simulink model "My_Model"  (R2022a)
settings: Solver=VariableStepAuto  StartTime=0.0  StopTime=10.0  RelTol=1e-3
libraries: neural x1294, spsSeriesRLCBranchLib x16, spsDiodeLib x14, spsMosfetLib x9, spsVoltageMeasurementLib x9, powerlib_extras x8, spsThreePhaseVIMeasurementLib x7, spsCurrentMeasurementLib x4, spsPVArrayLib x4, spsPWMGeneratorDCDCLib x4, spsTHDLib x4, spsThreePhaseParallelRLCBranchLib x3
(part 41 of 41)

== system My_Model/VSC Control/Current Regulator/7 layer network/Layer 6/LW{6,4} ==
  "ad{6,4}" : Inport  PortDimensions=25
      mask Display: e = 0.06;c1 = [120 230 180]/255;c2 = ([120 230 180]+0)/(256+128);c3 = ([120 230 180]+128)/(256+128);patch([0 1 1 0],[0 0 1 1],c1);patch([0 1 1 1-e 1-e 0+e],[0 0 1 1-e 0+e 0+e],c2);patch([0 0 1 1-e 0+e 0+e],[0 1 1 1-e 1-e 0+e],c3);plot([0 1 1 0 0],[0 0 1 1 0]);
  "IW{6,4}(1,:)'" : Constant  Value=[-0.377172170865255840244145701944944448769092559814453125;0.2166215985231878249361869848144124262034893035888671875;-0.8493855795188680612994858165620826184749603271484375;0.43917994402737026149452503887005150318145751953125;0.9925973529188081290186573824030347168445587158203125;0.52191832200732390933950455291778780519962310791015625;0.54353768542801095264849209343083202838897705078125;0.275162210381826144445227555479505099356174468994140625;0.81569668151233631903096465975977480411529541015625;-0.93565711696775666350589517605840228497982025146484375;-0.95509797101199678248661939505836926400661468505859375;0.09267489111664718726135703263935283757746219635009765625;-0.957854254009712580142377191805280745029449462890625;0.9681511422261415145129603843088261783123016357421875;0.59514371716452518779050251396256498992443084716796875;0.752293859537388254210554805467836558818817138671875;0.71189958405266562380120376474224030971527099609375;0.43163356736211000441727492216159589588642120361328125;-0.48098452705637051440845652905409224331378936767578125;-0.5182102404330437561696953707723878324031829833984375;-0.76663173461491995741567961886175908148288726806640625;0.920833310401809601586364806280471384525299072265625;-0.470710370173132275350980080474982969462871551513671875;-0.291630162894867428491352256969548761844635009765625;-0.363147996214426560523946818648255430161952972412109375]
      mask Display: e = 0.06;c1 = [120 150 230]/255;c2 = ([120 150 230]+0)/383;c3 = ([120 150 230]+128)/383;patch([0 1 1 0],[0 0 1 1],c1);patch([0 1 1 1-e 1-e 0+e],[0 0 1 1-e 0+e 0+e],c2);patch([0 0 1 1-e 0+e 0+e],[0 1 1 1-e 1-e 0+e],c3);plot([0 1 1 0 0],[0 0 1 1 0]);disp('weights');
  "IW{6,4}(2,:)'" : Constant  Value=[0.28732507639288284995160438484163023531436920166015625;-0.10063068272491536292445601930012344382703304290771484375;-0.07588109417358383790297438054039957933127880096435546875;0.8685538436173725340694318219902925193309783935546875;0.6786737694400650777737382668419741094112396240234375;0.034625140595084556716098944662007852457463741302490234375;-0.283134669546071748857940519883413799107074737548828125;0.08902086054486742228153417499925126321613788604736328125;-1.0830744519321864327565663188579492270946502685546875;0.1886613708921636434201474230576422996819019317626953125;0.71261338952339248198342147588846273720264434814453125;0.481217533055725843471606140155927278101444244384765625;0.311161297820213011977585892964270897209644317626953125;0.04995362741111118720649386659715673886239528656005859375;0.94351257987673953220308931122417561709880828857421875;0.66959181319910410223883445723913609981536865234375;0.7286748401637630490057517818058840930461883544921875;0.693751372005718902613580212346278131008148193359375;0.429237930795354827306908873651991598308086395263671875;0.432163392727505757395789487418369390070438385009765625;0.19340272304600369945859483777894638478755950927734375;-0.0179994719843084016730472285416908562183380126953125;1.1024282588912923674939747797907330095767974853515625;-0.413702287461697515436043204317684285342693328857421875;0.9039180203867420715369007666595280170440673828125]
      mask Display: e = 0.06;c1 = [120 150 230]/255;c2 = ([120 150 230]+0)/383;c3 = ([120 150 230]+128)/383;patch([0 1 1 0],[0 0 1 1],c1);patch([0 1 1 1-e 1-e 0+e],[0 0 1 1-e 0+e 0+e],c2);patch([0 0 1 1-e 0+e 0+e],[0 1 1 1-e 1-e 0+e],c3);plot([0 1 1 0 0],[0 0 1 1 0]);disp('weights');
  "IW{6,4}(3,:)'" : Constant  Value=[-0.64629750703306065862108198416535742580890655517578125;-1.098756912740348479218255306477658450603485107421875;-0.08866746573161542188667993968920200131833553314208984375;-1.07761686120664013088799038087017834186553955078125;-0.08707633180751157830901121315037016756832599639892578125;-0.69038565434756959948714438723982311785221099853515625;1.0878215450123225327416776053723879158496856689453125;0.35531945282508503591856197090237401425838470458984375;-0.469159418146348039524440309833153150975704193115234375;0.3372642338873126366394217257038690149784088134765625;0.08822785475541576605262861221490311436355113983154296875;1.1142599806591240163555767139769159257411956787109375;0.72730830477476182682750049934838898479938507080078125;1.0873952419514834044633744269958697259426116943359375;0.69099352817197712273156184892286546528339385986328125;-0.53374420227049845788513948718900792300701141357421875;0.1658638052207602464616087445392622612416744232177734375;-0.11318910522164206400308472666438319720327854156494140625;0.97839969428519679706113265638123266398906707763671875;-0.88106106612810630718257698390516452491283416748046875;-1.0220826746153062192234983740490861237049102783203125;0.3896164522899236981601234219851903617382049560546875;-1.0826724324468883775551830694894306361675262451171875;-0.87968776248958013841416914146975614130496978759765625;-0.0002833283639702526002235316582300583831965923309326171875]
      mask Display: e = 0.06;c1 = [120 150 230]/255;c2 = ([120 150 230]+0)/383;c3 = ([120 150 230]+128)/383;patch([0 1 1 0],[0 0 1 1],c1);patch([0 1 1 1-e 1-e 0+e],[0 0 1 1-e 0+e 0+e],c2);patch([0 0 1 1-e 0+e 0+e],[0 1 1 1-e 1-e 0+e],c3);plot([0 1 1 0 0],[0 0 1 1 0]);disp('weights');
  "IW{6,4}(4,:)'" : Constant  Value=[0.1890485194098358856518160564519348554313182830810546875;0.0216342621174379808046683848488100920803844928741455078125;0.12011949005118673083902791631771833635866641998291015625;-0.7077852872841623455002491027698852121829986572265625;-0.422049459183063968570337465280317701399326324462890625;-0.1909842843294208003523948491420014761388301849365234375;-1.1988173017738776859886229431140236556529998779296875;0.556276063052497438121690720436163246631622314453125;-0.79012741190201729590825152627076022326946258544921875;0.3767786001003521345609215131844393908977508544921875;0.4643024120214291894370717272977344691753387451171875;-0.1428330266733211229013278398269903846085071563720703125;0.468537774485975722082997663164860568940639495849609375;-1.0556031236689114027882396840141154825687408447265625;-0.50465636007393721573777156663709320127964019775390625;-0.67913261552524406550190860798466019332408905029296875;0.172008584272319298147380095542757771909236907958984375;-0.144475965090768265763898625664296559989452362060546875;1.001598299104828004857381529291160404682159423828125;-0.93051931461395931410862658594851382076740264892578125;0.796164649884228747822589866700582206249237060546875;0.96609541574008073183676970074884593486785888671875;-0.440361911057138843972325048525817692279815673828125;1.01609392982572810382180250599049031734466552734375;0.28456750588627055531532050736132077872753143310546875]
      mask Display: e = 0.06;c1 = [120 150 230]/255;c2 = ([120 150 230]+0)/383;c3 = ([120 150 230]+128)/383;patch([0 1 1 0],[0 0 1 1],c1);patch([0 1 1 1-e 1-e 0+e],[0 0 1 1-e 0+e 0+e],c2);patch([0 0 1 1-e 0+e 0+e],[0 1 1 1-e 1-e 0+e],c3);plot([0 1 1 0 0],[0 0 1 1 0]);disp('weights');
  "IW{6,4}(5,:)'" : Constant  Value=[0.27105149658062133166680496287881396710872650146484375;-0.193023461694903641916454262172919698059558868408203125;0.7128488109947801465438033119426108896732330322265625;-0.07239340949961368953946561077827936969697475433349609375;-0.9830308857488956331138751920661889016628265380859375;-0.7342459118544735208189422337454743683338165283203125;0.76633670396205888497576097506680525839328765869140625;-0.91777628549413592384809135182877071201801300048828125;0.99199765136458928349583175076986663043498992919921875;0.86263812078303647723487301846034824848175048828125;-0.642325683690944782000542545574717223644256591796875;-0.92113551914019320410176305813365615904331207275390625;-0.322276526479408131908854784342111088335514068603515625;-0.66431651873548169806582563978736288845539093017578125;-0.781701747176127614835650092572905123233795166015625;-0.39731852184941807148987891196156851947307586669921875;-0.461111000145560334662064860822283662855625152587890625;-0.059668897380601833291269286974056740291416645050048828125;0.55032218363215446021996513081830926239490509033203125;-0.70264903726413774354142560696345753967761993408203125;0.50662619166864775177572255415725521743297576904296875;0.09871715719628242069472179309741477482020854949951171875;1.0938888762767418061372381998808123171329498291015625;-0.80978778041068510962219306748011149466037750244140625;0.1924043984401257734173640301378327421844005584716796875]
      mask Display: e = 0.06;c1 = [120 150 230]/255;c2 = ([120 150 230]+0)/383;c3 = ([120 150 230]+128)/383;patch([0 1 1 0],[0 0 1 1],c1);patch([0 1 1 1-e 1-e 0+e],[0 0 1 1-e 0+e 0+e],c2);patch([0 0 1 1-e 0+e 0+e],[0 1 1 1-e 1-e 0+e],c3);plot([0 1 1 0 0],[0 0 1 1 0]);disp('weights');
  Mux : Mux  Inputs=5
      mask Display: e = 0.06;c1 = [120 150 230]/255;c2 = ([120 150 230]+0)/383;c3 = ([120 150 230]+128)/383;patch([0 1 1 0],[0 0 1 1],c1);patch([0 1 1 1-e 1-e 0+e],[0 0 1 1-e 0+e 0+e],c2);patch([0 0 1 1-e 0+e 0+e],[0 1 1 1-e 1-e 0+e],c3);plot([0 1 1 0 0],[0 0 1 1 0]);disp('Mux');
  dotprod{1..5} (5 alike) : neural/Weight Functions/dotprod
  "lz{6,4}" : Outport
      mask Display: e = 0.06;c1 = [120 230 180]/255;c2 = ([120 230 180]+0)/(256+128);c3 = ([120 230 180]+128)/(256+128);patch([0 1 1 0],[0 0 1 1],c1);patch([0 1 1 1-e 1-e 0+e],[0 0 1 1-e 0+e 0+e],c2);patch([0 0 1 1-e 0+e 0+e],[0 1 1 1-e 1-e 0+e],c3);plot([0 1 1 0 0],[0 0 1 1 0]);
  wires:
  "IW{6,4}(1,:)'"/1 -> dotprod1/1
  "ad{6,4}"/1 -> dotprod1/2, dotprod2/2, dotprod3/2, dotprod4/2, dotprod5/2
  dotprod1/1 -> Mux/1
  "IW{6,4}(2,:)'"/1 -> dotprod2/1
  dotprod2/1 -> Mux/2
  "IW{6,4}(3,:)'"/1 -> dotprod3/1
  dotprod3/1 -> Mux/3
  "IW{6,4}(4,:)'"/1 -> dotprod4/1
  dotprod4/1 -> Mux/4
  "IW{6,4}(5,:)'"/1 -> dotprod5/1
  dotprod5/1 -> Mux/5
  Mux/1 -> "lz{6,4}"/1

== system My_Model/VSC Control/Current Regulator/7 layer network/Layer 6/LW{6,5} ==
  "ad{6,5}" : Inport  PortDimensions=10
      mask Display: e = 0.06;c1 = [120 230 180]/255;c2 = ([120 230 180]+0)/(256+128);c3 = ([120 230 180]+128)/(256+128);patch([0 1 1 0],[0 0 1 1],c1);patch([0 1 1 1-e 1-e 0+e],[0 0 1 1-e 0+e 0+e],c2);patch([0 0 1 1-e 0+e 0+e],[0 1 1 1-e 1-e 0+e],c3);plot([0 1 1 0 0],[0 0 1 1 0]);
  "IW{6,5}(1,:)'" : Constant  Value=[0.429687815971328934683270972527679987251758575439453125;-0.346068629113729875346194830854074098169803619384765625;-0.98219313699815113949398437398485839366912841796875;-0.83739498807844869876504390049376524984836578369140625;-0.7885264055381722148041490072500891983509063720703125;-0.8543528519776548701969431931502185761928558349609375;0.035004635751464806270316643121986999176442623138427734375;-1.039210679049491492520473912009038031101226806640625;0.34006931875280965726915383129380643367767333984375;-0.502979274986845581452143960632383823394775390625]
      mask Display: e = 0.06;c1 = [120 150 230]/255;c2 = ([120 150 230]+0)/383;c3 = ([120 150 230]+128)/383;patch([0 1 1 0],[0 0 1 1],c1);patch([0 1 1 1-e 1-e 0+e],[0 0 1 1-e 0+e 0+e],c2);patch([0 0 1 1-e 0+e 0+e],[0 1 1 1-e 1-e 0+e],c3);plot([0 1 1 0 0],[0 0 1 1 0]);disp('weights');
  "IW{6,5}(2,:)'" : Constant  Value=[-1.0710077128761394948952556660515256226062774658203125;0.80353619826974165274435790706775151193141937255859375;-0.98744244173064676939333139671362005174160003662109375;0.68583647556494942154614591345307417213916778564453125;0.6769723731389734044938677470781840384006500244140625;0.8110004105230468329779114355915226042270660400390625;-0.38681250645933251686159337623394094407558441162109375;1.0558527284464924722584555638604797422885894775390625;-0.481185456649400100648250599988386966288089752197265625;0.56609801374014845354309954927884973585605621337890625]
      mask Display: e = 0.06;c1 = [120 150 230]/255;c2 = ([120 150 230]+0)/383;c3 = ([120 150 230]+128)/383;patch([0 1 1 0],[0 0 1 1],c1);patch([0 1 1 1-e 1-e 0+e],[0 0 1 1-e 0+e 0+e],c2);patch([0 0 1 1-e 0+e 0+e],[0 1 1 1-e 1-e 0+e],c3);plot([0 1 1 0 0],[0 0 1 1 0]);disp('weights');
  "IW{6,5}(3,:)'" : Constant  Value=[0.06271534584953468438595081124731223098933696746826171875;-0.57758435101291649704791097974521107971668243408203125;-1.1214217969680639885865502947126515209674835205078125;0.287195615160836414947453931745258159935474395751953125;-0.9518543521969726750597828868194483220577239990234375;0.49129271852601552605932511141872964799404144287109375;0.39119008942367405889939391272491775453090667724609375;1.1269337522951523578029764394159428775310516357421875;0.60893532118659077223554731972399167716503143310546875;0.9641221714535419540226257595350034534931182861328125]
      mask Display: e = 0.06;c1 = [120 150 230]/255;c2 = ([120 150 230]+0)/383;c3 = ([120 150 230]+128)/383;patch([0 1 1 0],[0 0 1 1],c1);patch([0 1 1 1-e 1-e 0+e],[0 0 1 1-e 0+e 0+e],c2);patch([0 0 1 1-e 0+e 0+e],[0 1 1 1-e 1-e 0+e],c3);plot([0 1 1 0 0],[0 0 1 1 0]);disp('weights');
  "IW{6,5}(4,:)'" : Constant  Value=[-1.158415351011949478987617112579755485057830810546875;0.1915558214143078530344865839651902206242084503173828125;0.444350035799105536060693566469126380980014801025390625;-1.0584621783405434580771498076501302421092987060546875;-0.6575764228372922293175406593945808708667755126953125;0.57266541551685989919207031562109477818012237548828125;-0.9518889867230029278033498485456220805644989013671875;-0.92910349289341065404101982494466938078403472900390625;0.13672757324302164949614279976231046020984649658203125;0.557587726090502666664860953460447490215301513671875]
      mask Display: e = 0.06;c1 = [120 150 230]/255;c2 = ([120 150 230]+0)/383;c3 = ([120 150 230]+128)/383;patch([0 1 1 0],[0 0 1 1],c1);patch([0 1 1 1-e 1-e 0+e],[0 0 1 1-e 0+e 0+e],c2);patch([0 0 1 1-e 0+e 0+e],[0 1 1 1-e 1-e 0+e],c3);plot([0 1 1 0 0],[0 0 1 1 0]);disp('weights');
  "IW{6,5}(5,:)'" : Constant  Value=[0.74460524721355880739537269619177095592021942138671875;0.99773442819647539803185054552159272134304046630859375;0.212480488677939838293440288907731883227825164794921875;-0.97662617042054578053722480035503394901752471923828125;-0.56627909108300344964703754158108495175838470458984375;0.341773472356023566565141891260282136499881744384765625;-0.79744639055360144741513295230106450617313385009765625;-0.0739957191774893996427664433213067241013050079345703125;-0.1541052068468630464881385933040292002260684967041015625;-0.1981364354380889258866460522767738439142704010009765625]
      mask Display: e = 0.06;c1 = [120 150 230]/255;c2 = ([120 150 230]+0)/383;c3 = ([120 150 230]+128)/383;patch([0 1 1 0],[0 0 1 1],c1);patch([0 1 1 1-e 1-e 0+e],[0 0 1 1-e 0+e 0+e],c2);patch([0 0 1 1-e 0+e 0+e],[0 1 1 1-e 1-e 0+e],c3);plot([0 1 1 0 0],[0 0 1 1 0]);disp('weights');
  Mux : Mux  Inputs=5
      mask Display: e = 0.06;c1 = [120 150 230]/255;c2 = ([120 150 230]+0)/383;c3 = ([120 150 230]+128)/383;patch([0 1 1 0],[0 0 1 1],c1);patch([0 1 1 1-e 1-e 0+e],[0 0 1 1-e 0+e 0+e],c2);patch([0 0 1 1-e 0+e 0+e],[0 1 1 1-e 1-e 0+e],c3);plot([0 1 1 0 0],[0 0 1 1 0]);disp('Mux');
  dotprod{1..5} (5 alike) : neural/Weight Functions/dotprod
  "lz{6,5}" : Outport
      mask Display: e = 0.06;c1 = [120 230 180]/255;c2 = ([120 230 180]+0)/(256+128);c3 = ([120 230 180]+128)/(256+128);patch([0 1 1 0],[0 0 1 1],c1);patch([0 1 1 1-e 1-e 0+e],[0 0 1 1-e 0+e 0+e],c2);patch([0 0 1 1-e 0+e 0+e],[0 1 1 1-e 1-e 0+e],c3);plot([0 1 1 0 0],[0 0 1 1 0]);
  wires:
  "IW{6,5}(1,:)'"/1 -> dotprod1/1
  "ad{6,5}"/1 -> dotprod1/2, dotprod2/2, dotprod3/2, dotprod4/2, dotprod5/2
  dotprod1/1 -> Mux/1
  "IW{6,5}(2,:)'"/1 -> dotprod2/1
  dotprod2/1 -> Mux/2
  "IW{6,5}(3,:)'"/1 -> dotprod3/1
  dotprod3/1 -> Mux/3
  "IW{6,5}(4,:)'"/1 -> dotprod4/1
  dotprod4/1 -> Mux/4
  "IW{6,5}(5,:)'"/1 -> dotprod5/1
  dotprod5/1 -> Mux/5
  Mux/1 -> "lz{6,5}"/1

== system My_Model/VSC Control/Current Regulator/7 layer network/Layer 7/Delays 1 ==
  "p{7}" : Inport  PortDimensions=2
      mask Display: e = 0.06;c1 = [120 230 180]/255;c2 = ([120 230 180]+0)/(256+128);c3 = ([120 230 180]+128)/(256+128);patch([0 1 1 0],[0 0 1 1],c1);patch([0 1 1 1-e 1-e 0+e],[0 0 1 1-e 0+e 0+e],c2);patch([0 0 1 1-e 0+e 0+e],[0 1 1 1-e 1-e 0+e],c3);plot([0 1 1 0 0],[0 0 1 1 0]);
  mux : Mux  Inputs=1
      mask Display: e = 0.06;c1 = [120 150 230]/255;c2 = ([120 150 230]+0)/383;c3 = ([120 150 230]+128)/383;patch([0 1 1 0],[0 0 1 1],c1);patch([0 1 1 1-e 1-e 0+e],[0 0 1 1-e 0+e 0+e],c2);patch([0 0 1 1-e 0+e 0+e],[0 1 1 1-e 1-e 0+e],c3);plot([0 1 1 0 0],[0 0 1 1 0]);disp('Mux')
  "pd{7,1}" : Outport
      mask Display: e = 0.06;c1 = [120 230 180]/255;c2 = ([120 230 180]+0)/(256+128);c3 = ([120 230 180]+128)/(256+128);patch([0 1 1 0],[0 0 1 1],c1);patch([0 1 1 1-e 1-e 0+e],[0 0 1 1-e 0+e 0+e],c2);patch([0 0 1 1-e 0+e 0+e],[0 1 1 1-e 1-e 0+e],c3);plot([0 1 1 0 0],[0 0 1 1 0]);
  wires:
  "p{7}"/1 -> mux/1
  mux/1 -> "pd{7,1}"/1

== system My_Model/VSC Control/Current Regulator/7 layer network/Layer 7/Delays 2 ==
  "p{7}" : Inport  PortDimensions=5
      mask Display: e = 0.06;c1 = [120 230 180]/255;c2 = ([120 230 180]+0)/(256+128);c3 = ([120 230 180]+128)/(256+128);patch([0 1 1 0],[0 0 1 1],c1);patch([0 1 1 1-e 1-e 0+e],[0 0 1 1-e 0+e 0+e],c2);patch([0 0 1 1-e 0+e 0+e],[0 1 1 1-e 1-e 0+e],c3);plot([0 1 1 0 0],[0 0 1 1 0]);
  mux : Mux  Inputs=1
      mask Display: e = 0.06;c1 = [120 150 230]/255;c2 = ([120 150 230]+0)/383;c3 = ([120 150 230]+128)/383;patch([0 1 1 0],[0 0 1 1],c1);patch([0 1 1 1-e 1-e 0+e],[0 0 1 1-e 0+e 0+e],c2);patch([0 0 1 1-e 0+e 0+e],[0 1 1 1-e 1-e 0+e],c3);plot([0 1 1 0 0],[0 0 1 1 0]);disp('Mux')
  "pd{7,1}" : Outport
      mask Display: e = 0.06;c1 = [120 230 180]/255;c2 = ([120 230 180]+0)/(256+128);c3 = ([120 230 180]+128)/(256+128);patch([0 1 1 0],[0 0 1 1],c1);patch([0 1 1 1-e 1-e 0+e],[0 0 1 1-e 0+e 0+e],c2);patch([0 0 1 1-e 0+e 0+e],[0 1 1 1-e 1-e 0+e],c3);plot([0 1 1 0 0],[0 0 1 1 0]);
  wires:
  "p{7}"/1 -> mux/1
  mux/1 -> "pd{7,1}"/1

== system My_Model/VSC Control/Current Regulator/7 layer network/Layer 7/Delays 3 ==
  "p{7}" : Inport  PortDimensions=10
      mask Display: e = 0.06;c1 = [120 230 180]/255;c2 = ([120 230 180]+0)/(256+128);c3 = ([120 230 180]+128)/(256+128);patch([0 1 1 0],[0 0 1 1],c1);patch([0 1 1 1-e 1-e 0+e],[0 0 1 1-e 0+e 0+e],c2);patch([0 0 1 1-e 0+e 0+e],[0 1 1 1-e 1-e 0+e],c3);plot([0 1 1 0 0],[0 0 1 1 0]);
  mux : Mux  Inputs=1
      mask Display: e = 0.06;c1 = [120 150 230]/255;c2 = ([120 150 230]+0)/383;c3 = ([120 150 230]+128)/383;patch([0 1 1 0],[0 0 1 1],c1);patch([0 1 1 1-e 1-e 0+e],[0 0 1 1-e 0+e 0+e],c2);patch([0 0 1 1-e 0+e 0+e],[0 1 1 1-e 1-e 0+e],c3);plot([0 1 1 0 0],[0 0 1 1 0]);disp('Mux')
  "pd{7,2}" : Outport
      mask Display: e = 0.06;c1 = [120 230 180]/255;c2 = ([120 230 180]+0)/(256+128);c3 = ([120 230 180]+128)/(256+128);patch([0 1 1 0],[0 0 1 1],c1);patch([0 1 1 1-e 1-e 0+e],[0 0 1 1-e 0+e 0+e],c2);patch([0 0 1 1-e 0+e 0+e],[0 1 1 1-e 1-e 0+e],c3);plot([0 1 1 0 0],[0 0 1 1 0]);
  wires:
  "p{7}"/1 -> mux/1
  mux/1 -> "pd{7,2}"/1

== system My_Model/VSC Control/Current Regulator/7 layer network/Layer 7/Delays 4 ==
  "p{7}" : Inport  PortDimensions=20
      mask Display: e = 0.06;c1 = [120 230 180]/255;c2 = ([120 230 180]+0)/(256+128);c3 = ([120 230 180]+128)/(256+128);patch([0 1 1 0],[0 0 1 1],c1);patch([0 1 1 1-e 1-e 0+e],[0 0 1 1-e 0+e 0+e],c2);patch([0 0 1 1-e 0+e 0+e],[0 1 1 1-e 1-e 0+e],c3);plot([0 1 1 0 0],[0 0 1 1 0]);
  mux : Mux  Inputs=1
      mask Display: e = 0.06;c1 = [120 150 230]/255;c2 = ([120 150 230]+0)/383;c3 = ([120 150 230]+128)/383;patch([0 1 1 0],[0 0 1 1],c1);patch([0 1 1 1-e 1-e 0+e],[0 0 1 1-e 0+e 0+e],c2);patch([0 0 1 1-e 0+e 0+e],[0 1 1 1-e 1-e 0+e],c3);plot([0 1 1 0 0],[0 0 1 1 0]);disp('Mux')
  "pd{7,3}" : Outport
      mask Display: e = 0.06;c1 = [120 230 180]/255;c2 = ([120 230 180]+0)/(256+128);c3 = ([120 230 180]+128)/(256+128);patch([0 1 1 0],[0 0 1 1],c1);patch([0 1 1 1-e 1-e 0+e],[0 0 1 1-e 0+e 0+e],c2);patch([0 0 1 1-e 0+e 0+e],[0 1 1 1-e 1-e 0+e],c3);plot([0 1 1 0 0],[0 0 1 1 0]);
  wires:
  "p{7}"/1 -> mux/1
  mux/1 -> "pd{7,3}"/1

== system My_Model/VSC Control/Current Regulator/7 layer network/Layer 7/Delays 5 ==
  "p{7}" : Inport  PortDimensions=25
      mask Display: e = 0.06;c1 = [120 230 180]/255;c2 = ([120 230 180]+0)/(256+128);c3 = ([120 230 180]+128)/(256+128);patch([0 1 1 0],[0 0 1 1],c1);patch([0 1 1 1-e 1-e 0+e],[0 0 1 1-e 0+e 0+e],c2);patch([0 0 1 1-e 0+e 0+e],[0 1 1 1-e 1-e 0+e],c3);plot([0 1 1 0 0],[0 0 1 1 0]);
  mux : Mux  Inputs=1
      mask Display: e = 0.06;c1 = [120 150 230]/255;c2 = ([120 150 230]+0)/383;c3 = ([120 150 230]+128)/383;patch([0 1 1 0],[0 0 1 1],c1);patch([0 1 1 1-e 1-e 0+e],[0 0 1 1-e 0+e 0+e],c2);patch([0 0 1 1-e 0+e 0+e],[0 1 1 1-e 1-e 0+e],c3);plot([0 1 1 0 0],[0 0 1 1 0]);disp('Mux')
  "pd{7,4}" : Outport
      mask Display: e = 0.06;c1 = [120 230 180]/255;c2 = ([120 230 180]+0)/(256+128);c3 = ([120 230 180]+128)/(256+128);patch([0 1 1 0],[0 0 1 1],c1);patch([0 1 1 1-e 1-e 0+e],[0 0 1 1-e 0+e 0+e],c2);patch([0 0 1 1-e 0+e 0+e],[0 1 1 1-e 1-e 0+e],c3);plot([0 1 1 0 0],[0 0 1 1 0]);
  wires:
  "p{7}"/1 -> mux/1
  mux/1 -> "pd{7,4}"/1

== system My_Model/VSC Control/Current Regulator/7 layer network/Layer 7/Delays 6 ==
  "p{7}" : Inport  PortDimensions=10
      mask Display: e = 0.06;c1 = [120 230 180]/255;c2 = ([120 230 180]+0)/(256+128);c3 = ([120 230 180]+128)/(256+128);patch([0 1 1 0],[0 0 1 1],c1);patch([0 1 1 1-e 1-e 0+e],[0 0 1 1-e 0+e 0+e],c2);patch([0 0 1 1-e 0+e 0+e],[0 1 1 1-e 1-e 0+e],c3);plot([0 1 1 0 0],[0 0 1 1 0]);
  mux : Mux  Inputs=1
      mask Display: e = 0.06;c1 = [120 150 230]/255;c2 = ([120 150 230]+0)/383;c3 = ([120 150 230]+128)/383;patch([0 1 1 0],[0 0 1 1],c1);patch([0 1 1 1-e 1-e 0+e],[0 0 1 1-e 0+e 0+e],c2);patch([0 0 1 1-e 0+e 0+e],[0 1 1 1-e 1-e 0+e],c3);plot([0 1 1 0 0],[0 0 1 1 0]);disp('Mux')
  "pd{7,5}" : Outport
      mask Display: e = 0.06;c1 = [120 230 180]/255;c2 = ([120 230 180]+0)/(256+128);c3 = ([120 230 180]+128)/(256+128);patch([0 1 1 0],[0 0 1 1],c1);patch([0 1 1 1-e 1-e 0+e],[0 0 1 1-e 0+e 0+e],c2);patch([0 0 1 1-e 0+e 0+e],[0 1 1 1-e 1-e 0+e],c3);plot([0 1 1 0 0],[0 0 1 1 0]);
  wires:
  "p{7}"/1 -> mux/1
  mux/1 -> "pd{7,5}"/1

== system My_Model/VSC Control/Current Regulator/7 layer network/Layer 7/Delays 7 ==
  "p{7}" : Inport  PortDimensions=5
      mask Display: e = 0.06;c1 = [120 230 180]/255;c2 = ([120 230 180]+0)/(256+128);c3 = ([120 230 180]+128)/(256+128);patch([0 1 1 0],[0 0 1 1],c1);patch([0 1 1 1-e 1-e 0+e],[0 0 1 1-e 0+e 0+e],c2);patch([0 0 1 1-e 0+e 0+e],[0 1 1 1-e 1-e 0+e],c3);plot([0 1 1 0 0],[0 0 1 1 0]);
  mux : Mux  Inputs=1
      mask Display: e = 0.06;c1 = [120 150 230]/255;c2 = ([120 150 230]+0)/383;c3 = ([120 150 230]+128)/383;patch([0 1 1 0],[0 0 1 1],c1);patch([0 1 1 1-e 1-e 0+e],[0 0 1 1-e 0+e 0+e],c2);patch([0 0 1 1-e 0+e 0+e],[0 1 1 1-e 1-e 0+e],c3);plot([0 1 1 0 0],[0 0 1 1 0]);disp('Mux')
  "pd{7,6}" : Outport
      mask Display: e = 0.06;c1 = [120 230 180]/255;c2 = ([120 230 180]+0)/(256+128);c3 = ([120 230 180]+128)/(256+128);patch([0 1 1 0],[0 0 1 1],c1);patch([0 1 1 1-e 1-e 0+e],[0 0 1 1-e 0+e 0+e],c2);patch([0 0 1 1-e 0+e 0+e],[0 1 1 1-e 1-e 0+e],c3);plot([0 1 1 0 0],[0 0 1 1 0]);
  wires:
  "p{7}"/1 -> mux/1
  mux/1 -> "pd{7,6}"/1

== system My_Model/VSC Control/Current Regulator/7 layer network/Layer 7/IW{7,1} ==
  "pd{7,1}" : Inport  PortDimensions=2
      mask Display: e = 0.06;c1 = [120 230 180]/255;c2 = ([120 230 180]+0)/(256+128);c3 = ([120 230 180]+128)/(256+128);patch([0 1 1 0],[0 0 1 1],c1);patch([0 1 1 1-e 1-e 0+e],[0 0 1 1-e 0+e 0+e],c2);patch([0 0 1 1-e 0+e 0+e],[0 1 1 1-e 1-e 0+e],c3);plot([0 1 1 0 0],[0 0 1 1 0]);
  "IW{7,1}(1,:)'" : Constant  Value=[1.271226380744853390325488362577743828296661376953125;-0.017924339888765794537306419442757032811641693115234375]
      mask Display: e = 0.06;c1 = [120 150 230]/255;c2 = ([120 150 230]+0)/383;c3 = ([120 150 230]+128)/383;patch([0 1 1 0],[0 0 1 1],c1);patch([0 1 1 1-e 1-e 0+e],[0 0 1 1-e 0+e 0+e],c2);patch([0 0 1 1-e 0+e 0+e],[0 1 1 1-e 1-e 0+e],c3);plot([0 1 1 0 0],[0 0 1 1 0]);disp('Weights');
  "IW{7,1}(2,:)'" : Constant  Value=[-0.253325923879466008425964673733687959611415863037109375;0.752854052452355926305926914210431277751922607421875]
      mask Display: e = 0.06;c1 = [120 150 230]/255;c2 = ([120 150 230]+0)/383;c3 = ([120 150 230]+128)/383;patch([0 1 1 0],[0 0 1 1],c1);patch([0 1 1 1-e 1-e 0+e],[0 0 1 1-e 0+e 0+e],c2);patch([0 0 1 1-e 0+e 0+e],[0 1 1 1-e 1-e 0+e],c3);plot([0 1 1 0 0],[0 0 1 1 0]);disp('Weights');
  Mux : Mux  Inputs=2
      mask Display: e = 0.06;c1 = [120 150 230]/255;c2 = ([120 150 230]+0)/383;c3 = ([120 150 230]+128)/383;patch([0 1 1 0],[0 0 1 1],c1);patch([0 1 1 1-e 1-e 0+e],[0 0 1 1-e 0+e 0+e],c2);patch([0 0 1 1-e 0+e 0+e],[0 1 1 1-e 1-e 0+e],c3);plot([0 1 1 0 0],[0 0 1 1 0]);disp('Mux');
  dotprod1 : neural/Weight Functions/dotprod
  dotprod2 : neural/Weight Functions/dotprod
  "iz{7,1}" : Outport
      mask Display: e = 0.06;c1 = [120 230 180]/255;c2 = ([120 230 180]+0)/(256+128);c3 = ([120 230 180]+128)/(256+128);patch([0 1 1 0],[0 0 1 1],c1);patch([0 1 1 1-e 1-e 0+e],[0 0 1 1-e 0+e 0+e],c2);patch([0 0 1 1-e 0+e 0+e],[0 1 1 1-e 1-e 0+e],c3);plot([0 1 1 0 0],[0 0 1 1 0]);
  wires:
  "IW{7,1}(1,:)'"/1 -> dotprod1/1
  "pd{7,1}"/1 -> dotprod1/2, dotprod2/2
  dotprod1/1 -> Mux/1
  "IW{7,1}(2,:)'"/1 -> dotprod2/1
  dotprod2/1 -> Mux/2
  Mux/1 -> "iz{7,1}"/1

== system My_Model/VSC Control/Current Regulator/7 layer network/Layer 7/LW{7,1} ==
  "ad{7,1}" : Inport  PortDimensions=5
      mask Display: e = 0.06;c1 = [120 230 180]/255;c2 = ([120 230 180]+0)/(256+128);c3 = ([120 230 180]+128)/(256+128);patch([0 1 1 0],[0 0 1 1],c1);patch([0 1 1 1-e 1-e 0+e],[0 0 1 1-e 0+e 0+e],c2);patch([0 0 1 1-e 0+e 0+e],[0 1 1 1-e 1-e 0+e],c3);plot([0 1 1 0 0],[0 0 1 1 0]);
  "IW{7,1}(1,:)'" : Constant  Value=[-0.1399721419724498094883102794483420439064502716064453125;0.9169102476718442584768808956141583621501922607421875;-0.33071053243995873760496806426090188324451446533203125;-0.60184994233361199800214080823934637010097503662109375;0.58924366070781120097166194682358764111995697021484375]
      mask Display: e = 0.06;c1 = [120 150 230]/255;c2 = ([120 150 230]+0)/383;c3 = ([120 150 230]+128)/383;patch([0 1 1 0],[0 0 1 1],c1);patch([0 1 1 1-e 1-e 0+e],[0 0 1 1-e 0+e 0+e],c2);patch([0 0 1 1-e 0+e 0+e],[0 1 1 1-e 1-e 0+e],c3);plot([0 1 1 0 0],[0 0 1 1 0]);disp('weights');
  "IW{7,1}(2,:)'" : Constant  Value=[-0.5457231422189112723941661897697485983371734619140625;-0.57571827217991222713777688113623298704624176025390625;0.1647711432619676508171124851287459023296833038330078125;0.183526978590318912143430907235597260296344757080078125;0.0237926496519859191625112515566797810606658458709716796875]
      mask Display: e = 0.06;c1 = [120 150 230]/255;c2 = ([120 150 230]+0)/383;c3 = ([120 150 230]+128)/383;patch([0 1 1 0],[0 0 1 1],c1);patch([0 1 1 1-e 1-e 0+e],[0 0 1 1-e 0+e 0+e],c2);patch([0 0 1 1-e 0+e 0+e],[0 1 1 1-e 1-e 0+e],c3);plot([0 1 1 0 0],[0 0 1 1 0]);disp('weights');
  Mux : Mux  Inputs=2
      mask Display: e = 0.06;c1 = [120 150 230]/255;c2 = ([120 150 230]+0)/383;c3 = ([120 150 230]+128)/383;patch([0 1 1 0],[0 0 1 1],c1);patch([0 1 1 1-e 1-e 0+e],[0 0 1 1-e 0+e 0+e],c2);patch([0 0 1 1-e 0+e 0+e],[0 1 1 1-e 1-e 0+e],c3);plot([0 1 1 0 0],[0 0 1 1 0]);disp('Mux');
  dotprod1 : neural/Weight Functions/dotprod
  dotprod2 : neural/Weight Functions/dotprod
  "lz{7,1}" : Outport
      mask Display: e = 0.06;c1 = [120 230 180]/255;c2 = ([120 230 180]+0)/(256+128);c3 = ([120 230 180]+128)/(256+128);patch([0 1 1 0],[0 0 1 1],c1);patch([0 1 1 1-e 1-e 0+e],[0 0 1 1-e 0+e 0+e],c2);patch([0 0 1 1-e 0+e 0+e],[0 1 1 1-e 1-e 0+e],c3);plot([0 1 1 0 0],[0 0 1 1 0]);
  wires:
  "IW{7,1}(1,:)'"/1 -> dotprod1/1
  "ad{7,1}"/1 -> dotprod1/2, dotprod2/2
  dotprod1/1 -> Mux/1
  "IW{7,1}(2,:)'"/1 -> dotprod2/1
  dotprod2/1 -> Mux/2
  Mux/1 -> "lz{7,1}"/1

== system My_Model/VSC Control/Current Regulator/7 layer network/Layer 7/LW{7,2} ==
  "ad{7,2}" : Inport  PortDimensions=10
      mask Display: e = 0.06;c1 = [120 230 180]/255;c2 = ([120 230 180]+0)/(256+128);c3 = ([120 230 180]+128)/(256+128);patch([0 1 1 0],[0 0 1 1],c1);patch([0 1 1 1-e 1-e 0+e],[0 0 1 1-e 0+e 0+e],c2);patch([0 0 1 1-e 0+e 0+e],[0 1 1 1-e 1-e 0+e],c3);plot([0 1 1 0 0],[0 0 1 1 0]);
  "IW{7,2}(1,:)'" : Constant  Value=[0.295330180327427083142310948460362851619720458984375;-0.5251128972157454999347692137234844267368316650390625;-0.7180734971715343473164239185280166566371917724609375;0.5919270243185563717958075358183123171329498291015625;0.11953399765489790274042292139711207710206508636474609375;0.342647990599721563587110040316474623978137969970703125;-0.0159771387543272691544871122459881007671356201171875;-0.704647027112888846289706634706817567348480224609375;-0.091153538469831374424501291287015192210674285888671875;-0.157429755972143536890683890305808745324611663818359375]
      mask Display: e = 0.06;c1 = [120 150 230]/255;c2 = ([120 150 230]+0)/383;c3 = ([120 150 230]+128)/383;patch([0 1 1 0],[0 0 1 1],c1);patch([0 1 1 1-e 1-e 0+e],[0 0 1 1-e 0+e 0+e],c2);patch([0 0 1 1-e 0+e 0+e],[0 1 1 1-e 1-e 0+e],c3);plot([0 1 1 0 0],[0 0 1 1 0]);disp('weights');
  "IW{7,2}(2,:)'" : Constant  Value=[0.65692183983364749177980002059484831988811492919921875;0.2333722687588110911161010108116897754371166229248046875;0.040390642172835687639942392479497357271611690521240234375;0.7737311897419905104555937214172445237636566162109375;-0.309691966896001591447173950655269436538219451904296875;0.66971479097063635332887088225106708705425262451171875;1.0306742930276191483329739639884792268276214599609375;-0.59097725639540066300270382271264679729938507080078125;0.0019314451221247551371273942777406773529946804046630859375;-0.336081037894097656160141696091159246861934661865234375]
      mask Display: e = 0.06;c1 = [120 150 230]/255;c2 = ([120 150 230]+0)/383;c3 = ([120 150 230]+128)/383;patch([0 1 1 0],[0 0 1 1],c1);patch([0 1 1 1-e 1-e 0+e],[0 0 1 1-e 0+e 0+e],c2);patch([0 0 1 1-e 0+e 0+e],[0 1 1 1-e 1-e 0+e],c3);plot([0 1 1 0 0],[0 0 1 1 0]);disp('weights');
  Mux : Mux  Inputs=2
      mask Display: e = 0.06;c1 = [120 150 230]/255;c2 = ([120 150 230]+0)/383;c3 = ([120 150 230]+128)/383;patch([0 1 1 0],[0 0 1 1],c1);patch([0 1 1 1-e 1-e 0+e],[0 0 1 1-e 0+e 0+e],c2);patch([0 0 1 1-e 0+e 0+e],[0 1 1 1-e 1-e 0+e],c3);plot([0 1 1 0 0],[0 0 1 1 0]);disp('Mux');
  dotprod1 : neural/Weight Functions/dotprod
  dotprod2 : neural/Weight Functions/dotprod
  "lz{7,2}" : Outport
      mask Display: e = 0.06;c1 = [120 230 180]/255;c2 = ([120 230 180]+0)/(256+128);c3 = ([120 230 180]+128)/(256+128);patch([0 1 1 0],[0 0 1 1],c1);patch([0 1 1 1-e 1-e 0+e],[0 0 1 1-e 0+e 0+e],c2);patch([0 0 1 1-e 0+e 0+e],[0 1 1 1-e 1-e 0+e],c3);plot([0 1 1 0 0],[0 0 1 1 0]);
  wires:
  "IW{7,2}(1,:)'"/1 -> dotprod1/1
  "ad{7,2}"/1 -> dotprod1/2, dotprod2/2
  dotprod1/1 -> Mux/1
  "IW{7,2}(2,:)'"/1 -> dotprod2/1
  dotprod2/1 -> Mux/2
  Mux/1 -> "lz{7,2}"/1

== system My_Model/VSC Control/Current Regulator/7 layer network/Layer 7/LW{7,3} ==
  "ad{7,3}" : Inport  PortDimensions=20
      mask Display: e = 0.06;c1 = [120 230 180]/255;c2 = ([120 230 180]+0)/(256+128);c3 = ([120 230 180]+128)/(256+128);patch([0 1 1 0],[0 0 1 1],c1);patch([0 1 1 1-e 1-e 0+e],[0 0 1 1-e 0+e 0+e],c2);patch([0 0 1 1-e 0+e 0+e],[0 1 1 1-e 1-e 0+e],c3);plot([0 1 1 0 0],[0 0 1 1 0]);
  "IW{7,3}(1,:)'" : Constant  Value=[0.20027745385358297625089107896201312541961669921875;-0.1260101494140383471265209891498670913279056549072265625;-0.52953910171273255169666072106338106095790863037109375;0.188971290437726036071097723834100179374217987060546875;-0.580890073741141321761460858397185802459716796875;-0.28614803792992937747641235546325333416461944580078125;0.66112637931677242786321357925771735608577728271484375;0.77887882743118230788326172842062078416347503662109375;0.486831181941093316112301181419752538204193115234375;0.86114110403958876727159577058046124875545501708984375;0.044924617629774767080252928508343757130205631256103515625;-0.60614986113057500727308024579542689025402069091796875;0.209005860819568234365561920640175230801105499267578125;-0.0200126231667867061914112269960241974331438541412353515625;0.0501942622388361348040319853680557571351528167724609375;-0.197770185894764971568093869791482575237751007080078125;-0.318301485194999178585106847094721160829067230224609375;-0.27003721063527053036779079775442369282245635986328125;0.0163002869066101452322214981904835440218448638916015625;0.383966415278070460903592220347491092979907989501953125]
      mask Display: e = 0.06;c1 = [120 150 230]/255;c2 = ([120 150 230]+0)/383;c3 = ([120 150 230]+128)/383;patch([0 1 1 0],[0 0 1 1],c1);patch([0 1 1 1-e 1-e 0+e],[0 0 1 1-e 0+e 0+e],c2);patch([0 0 1 1-e 0+e 0+e],[0 1 1 1-e 1-e 0+e],c3);plot([0 1 1 0 0],[0 0 1 1 0]);disp('weights');
  "IW{7,3}(2,:)'" : Constant  Value=[-0.76833057526552173133183032405213452875614166259765625;-0.407507852490404942624735440404037944972515106201171875;-0.6316340607881538726786629922571592032909393310546875;-0.436704666830578902558812615097849629819393157958984375;-0.9148923804842199469788965870975516736507415771484375;0.164047492017683815834772076414083130657672882080078125;-0.895651309274045015484944087802432477474212646484375;-0.79712907754279604954916749193216674029827117919921875;0.4675309509988478939845890636206604540348052978515625;-0.73113984888177385723651013904600404202938079833984375;-0.033513274236622370150229244245565496385097503662109375;0.1900732148990969816448881601900211535394191741943359375;-0.46971992213198798804540956552955321967601776123046875;1.0050656702436155942592677092761732637882232666015625;0.494955523701778032918952021645964123308658599853515625;-0.90838332320744574754911582203931175172328948974609375;0.492983457766519583831410500351921655237674713134765625;-0.83638405841522411865440744804800488054752349853515625;-0.267676691673026490025932844218914397060871124267578125;-0.092151028037154691929799810168333351612091064453125]
      mask Display: e = 0.06;c1 = [120 150 230]/255;c2 = ([120 150 230]+0)/383;c3 = ([120 150 230]+128)/383;patch([0 1 1 0],[0 0 1 1],c1);patch([0 1 1 1-e 1-e 0+e],[0 0 1 1-e 0+e 0+e],c2);patch([0 0 1 1-e 0+e 0+e],[0 1 1 1-e 1-e 0+e],c3);plot([0 1 1 0 0],[0 0 1 1 0]);disp('weights');
  Mux : Mux  Inputs=2
      mask Display: e = 0.06;c1 = [120 150 230]/255;c2 = ([120 150 230]+0)/383;c3 = ([120 150 230]+128)/383;patch([0 1 1 0],[0 0 1 1],c1);patch([0 1 1 1-e 1-e 0+e],[0 0 1 1-e 0+e 0+e],c2);patch([0 0 1 1-e 0+e 0+e],[0 1 1 1-e 1-e 0+e],c3);plot([0 1 1 0 0],[0 0 1 1 0]);disp('Mux');
  dotprod1 : neural/Weight Functions/dotprod
  dotprod2 : neural/Weight Functions/dotprod
  "lz{7,3}" : Outport
      mask Display: e = 0.06;c1 = [120 230 180]/255;c2 = ([120 230 180]+0)/(256+128);c3 = ([120 230 180]+128)/(256+128);patch([0 1 1 0],[0 0 1 1],c1);patch([0 1 1 1-e 1-e 0+e],[0 0 1 1-e 0+e 0+e],c2);patch([0 0 1 1-e 0+e 0+e],[0 1 1 1-e 1-e 0+e],c3);plot([0 1 1 0 0],[0 0 1 1 0]);
  wires:
  "IW{7,3}(1,:)'"/1 -> dotprod1/1
  "ad{7,3}"/1 -> dotprod1/2, dotprod2/2
  dotprod1/1 -> Mux/1
  "IW{7,3}(2,:)'"/1 -> dotprod2/1
  dotprod2/1 -> Mux/2
  Mux/1 -> "lz{7,3}"/1

== system My_Model/VSC Control/Current Regulator/7 layer network/Layer 7/LW{7,4} ==
  "ad{7,4}" : Inport  PortDimensions=25
      mask Display: e = 0.06;c1 = [120 230 180]/255;c2 = ([120 230 180]+0)/(256+128);c3 = ([120 230 180]+128)/(256+128);patch([0 1 1 0],[0 0 1 1],c1);patch([0 1 1 1-e 1-e 0+e],[0 0 1 1-e 0+e 0+e],c2);patch([0 0 1 1-e 0+e 0+e],[0 1 1 1-e 1-e 0+e],c3);plot([0 1 1 0 0],[0 0 1 1 0]);
  "IW{7,4}(1,:)'" : Constant  Value=[0.5058570630804475332098490980570204555988311767578125;-0.5874372523511517396599401763523928821086883544921875;0.56949788927491307166661727023893035948276519775390625;-0.7329802102713875999739912003860808908939361572265625;0.01470864083338267215561590006700498634018003940582275390625;0.2014852049501108244289326876241830177605152130126953125;0.6429554686248308836837850321899168193340301513671875;-0.78259660982451773048040877256426028907299041748046875;-0.397310699884527218639362899921252392232418060302734375;-0.352704493361016335750690586792188696563243865966796875;-0.641633092537038152158856973983347415924072265625;0.75467657027388035384518616410787217319011688232421875;0.311639130152457421996103903438779525458812713623046875;-0.080633552989745116423847548503545112907886505126953125;0.82530563178383620215328164704260416328907012939453125;-0.011532291273996346514518762660372885875403881072998046875;-0.396699630925869684006102033890783786773681640625;0.79295222559601008516239062373642809689044952392578125;-0.2421205129116431320479563282788149081170558929443359375;0.423902019551200270885971121970214881002902984619140625;0.74200788988278976177070944686420261859893798828125;-0.190550783943221835325942947747535072267055511474609375;0.5056309189908727574902513879351317882537841796875;-0.5744480109941723089406195867923088371753692626953125;0.08353998429143690007681044562559691257774829864501953125]
      mask Display: e = 0.06;c1 = [120 150 230]/255;c2 = ([120 150 230]+0)/383;c3 = ([120 150 230]+128)/383;patch([0 1 1 0],[0 0 1 1],c1);patch([0 1 1 1-e 1-e 0+e],[0 0 1 1-e 0+e 0+e],c2);patch([0 0 1 1-e 0+e 0+e],[0 1 1 1-e 1-e 0+e],c3);plot([0 1 1 0 0],[0 0 1 1 0]);disp('weights');
  "IW{7,4}(2,:)'" : Constant  Value=[0.488251138779681681523214820117573253810405731201171875;-0.68117271377829891054744848588597960770130157470703125;0.351341608031384478039171881391666829586029052734375;0.745459740084354560707424752763472497463226318359375;0.1585372494158440448419611357167013920843601226806640625;0.58847832459078908140526209535892121493816375732421875;-0.14206273580412120960403399294591508805751800537109375;0.442097263542864771235230136881000362336635589599609375;0.6838119313297716939104020639206282794475555419921875;0.49558243456121398029523561490350402891635894775390625;-0.83197428465458289625900079045095480978488922119140625;-0.85417296879087756256154762013466097414493560791015625;0.40793250382095980199892437667585909366607666015625;-0.26325006092149438874372435748227871954441070556640625;-0.2477478874782114981467628922473522834479808807373046875;-0.56607502203011250685449340380728244781494140625;-0.38032927310454278657658733209245838224887847900390625;-0.437073567609963353763902205173508264124393463134765625;0.14638534969418059983325974826584570109844207763671875;-0.69991665948476988745596827357076108455657958984375;-0.833780438172883719971650862134993076324462890625;-0.99113799510334110731690770990098826587200164794921875;0.469733003071002241934905896414420567452907562255859375;0.435069236968946004839864372115698643028736114501953125;0.670416154513647111201635198085568845272064208984375]
      mask Display: e = 0.06;c1 = [120 150 230]/255;c2 = ([120 150 230]+0)/383;c3 = ([120 150 230]+128)/383;patch([0 1 1 0],[0 0 1 1],c1);patch([0 1 1 1-e 1-e 0+e],[0 0 1 1-e 0+e 0+e],c2);patch([0 0 1 1-e 0+e 0+e],[0 1 1 1-e 1-e 0+e],c3);plot([0 1 1 0 0],[0 0 1 1 0]);disp('weights');
  Mux : Mux  Inputs=2
      mask Display: e = 0.06;c1 = [120 150 230]/255;c2 = ([120 150 230]+0)/383;c3 = ([120 150 230]+128)/383;patch([0 1 1 0],[0 0 1 1],c1);patch([0 1 1 1-e 1-e 0+e],[0 0 1 1-e 0+e 0+e],c2);patch([0 0 1 1-e 0+e 0+e],[0 1 1 1-e 1-e 0+e],c3);plot([0 1 1 0 0],[0 0 1 1 0]);disp('Mux');
  dotprod1 : neural/Weight Functions/dotprod
  dotprod2 : neural/Weight Functions/dotprod
  "lz{7,4}" : Outport
      mask Display: e = 0.06;c1 = [120 230 180]/255;c2 = ([120 230 180]+0)/(256+128);c3 = ([120 230 180]+128)/(256+128);patch([0 1 1 0],[0 0 1 1],c1);patch([0 1 1 1-e 1-e 0+e],[0 0 1 1-e 0+e 0+e],c2);patch([0 0 1 1-e 0+e 0+e],[0 1 1 1-e 1-e 0+e],c3);plot([0 1 1 0 0],[0 0 1 1 0]);
  wires:
  "IW{7,4}(1,:)'"/1 -> dotprod1/1
  "ad{7,4}"/1 -> dotprod1/2, dotprod2/2
  dotprod1/1 -> Mux/1
  "IW{7,4}(2,:)'"/1 -> dotprod2/1
  dotprod2/1 -> Mux/2
  Mux/1 -> "lz{7,4}"/1

== system My_Model/VSC Control/Current Regulator/7 layer network/Layer 7/LW{7,5} ==
  "ad{7,5}" : Inport  PortDimensions=10
      mask Display: e = 0.06;c1 = [120 230 180]/255;c2 = ([120 230 180]+0)/(256+128);c3 = ([120 230 180]+128)/(256+128);patch([0 1 1 0],[0 0 1 1],c1);patch([0 1 1 1-e 1-e 0+e],[0 0 1 1-e 0+e 0+e],c2);patch([0 0 1 1-e 0+e 0+e],[0 1 1 1-e 1-e 0+e],c3);plot([0 1 1 0 0],[0 0 1 1 0]);
  "IW{7,5}(1,:)'" : Constant  Value=[0.149413382095861912990386599631165154278278350830078125;-0.124041262389895046158727609508787281811237335205078125;-0.058866311741444611593809810301536344923079013824462890625;0.8824639568828518410015249173738993704319000244140625;-0.494351981371395188258333064368343912065029144287109375;0.304941699668616283958044732571579515933990478515625;-0.60881619944982923176013400734518654644489288330078125;0.167569540376651004986996440493385307490825653076171875;-0.5802696132914089144350100468727760016918182373046875;-0.038473931669981399628088780673351720906794071197509765625]
      mask Display: e = 0.06;c1 = [120 150 230]/255;c2 = ([120 150 230]+0)/383;c3 = ([120 150 230]+128)/383;patch([0 1 1 0],[0 0 1 1],c1);patch([0 1 1 1-e 1-e 0+e],[0 0 1 1-e 0+e 0+e],c2);patch([0 0 1 1-e 0+e 0+e],[0 1 1 1-e 1-e 0+e],c3);plot([0 1 1 0 0],[0 0 1 1 0]);disp('weights');
  "IW{7,5}(2,:)'" : Constant  Value=[0.78878855873790520991661878724698908627033233642578125;-0.085257555063405765505279987337416969239711761474609375;-0.2349016859477008056789060219671227969229221343994140625;-0.0302646459746021660730530555838413420133292675018310546875;-0.034947437716549421826695009940522140823304653167724609375;-0.175574313251335656360652137664146721363067626953125;0.7691024858569572852928786232951097190380096435546875;-0.25374571779057608633678455589688383042812347412109375;-0.6355860653613818467277951640426181256771087646484375;-0.1724689207237434518393826010651537217199802398681640625]
      mask Display: e = 0.06;c1 = [120 150 230]/255;c2 = ([120 150 230]+0)/383;c3 = ([120 150 230]+128)/383;patch([0 1 1 0],[0 0 1 1],c1);patch([0 1 1 1-e 1-e 0+e],[0 0 1 1-e 0+e 0+e],c2);patch([0 0 1 1-e 0+e 0+e],[0 1 1 1-e 1-e 0+e],c3);plot([0 1 1 0 0],[0 0 1 1 0]);disp('weights');
  Mux : Mux  Inputs=2
      mask Display: e = 0.06;c1 = [120 150 230]/255;c2 = ([120 150 230]+0)/383;c3 = ([120 150 230]+128)/383;patch([0 1 1 0],[0 0 1 1],c1);patch([0 1 1 1-e 1-e 0+e],[0 0 1 1-e 0+e 0+e],c2);patch([0 0 1 1-e 0+e 0+e],[0 1 1 1-e 1-e 0+e],c3);plot([0 1 1 0 0],[0 0 1 1 0]);disp('Mux');
  dotprod1 : neural/Weight Functions/dotprod
  dotprod2 : neural/Weight Functions/dotprod
  "lz{7,5}" : Outport
      mask Display: e = 0.06;c1 = [120 230 180]/255;c2 = ([120 230 180]+0)/(256+128);c3 = ([120 230 180]+128)/(256+128);patch([0 1 1 0],[0 0 1 1],c1);patch([0 1 1 1-e 1-e 0+e],[0 0 1 1-e 0+e 0+e],c2);patch([0 0 1 1-e 0+e 0+e],[0 1 1 1-e 1-e 0+e],c3);plot([0 1 1 0 0],[0 0 1 1 0]);
  wires:
  "IW{7,5}(1,:)'"/1 -> dotprod1/1
  "ad{7,5}"/1 -> dotprod1/2, dotprod2/2
  dotprod1/1 -> Mux/1
  "IW{7,5}(2,:)'"/1 -> dotprod2/1
  dotprod2/1 -> Mux/2
  Mux/1 -> "lz{7,5}"/1

== system My_Model/VSC Control/Current Regulator/7 layer network/Layer 7/LW{7,6} ==
  "ad{7,6}" : Inport  PortDimensions=5
      mask Display: e = 0.06;c1 = [120 230 180]/255;c2 = ([120 230 180]+0)/(256+128);c3 = ([120 230 180]+128)/(256+128);patch([0 1 1 0],[0 0 1 1],c1);patch([0 1 1 1-e 1-e 0+e],[0 0 1 1-e 0+e 0+e],c2);patch([0 0 1 1-e 0+e 0+e],[0 1 1 1-e 1-e 0+e],c3);plot([0 1 1 0 0],[0 0 1 1 0]);
  "IW{7,6}(1,:)'" : Constant  Value=[0.49279998153963033846736152554512955248355865478515625;0.59477852247353057979495360996224917471408843994140625;-0.76548132712853289572052517542033456265926361083984375;-0.62467527305143233373740940805873833596706390380859375;0.03763739447955920247590455574027146212756633758544921875]
      mask Display: e = 0.06;c1 = [120 150 230]/255;c2 = ([120 150 230]+0)/383;c3 = ([120 150 230]+128)/383;patch([0 1 1 0],[0 0 1 1],c1);patch([0 1 1 1-e 1-e 0+e],[0 0 1 1-e 0+e 0+e],c2);patch([0 0 1 1-e 0+e 0+e],[0 1 1 1-e 1-e 0+e],c3);plot([0 1 1 0 0],[0 0 1 1 0]);disp('weights');
  "IW{7,6}(2,:)'" : Constant  Value=[-0.85396983541003057549545474103069864213466644287109375;0.37430103311434892443543276385753415524959564208984375;0.72725564130029762832663209337624721229076385498046875;0.29639663136812555155330528577906079590320587158203125;-0.56651772196903082967622822252451442182064056396484375]
      mask Display: e = 0.06;c1 = [120 150 230]/255;c2 = ([120 150 230]+0)/383;c3 = ([120 150 230]+128)/383;patch([0 1 1 0],[0 0 1 1],c1);patch([0 1 1 1-e 1-e 0+e],[0 0 1 1-e 0+e 0+e],c2);patch([0 0 1 1-e 0+e 0+e],[0 1 1 1-e 1-e 0+e],c3);plot([0 1 1 0 0],[0 0 1 1 0]);disp('weights');
  Mux : Mux  Inputs=2
      mask Display: e = 0.06;c1 = [120 150 230]/255;c2 = ([120 150 230]+0)/383;c3 = ([120 150 230]+128)/383;patch([0 1 1 0],[0 0 1 1],c1);patch([0 1 1 1-e 1-e 0+e],[0 0 1 1-e 0+e 0+e],c2);patch([0 0 1 1-e 0+e 0+e],[0 1 1 1-e 1-e 0+e],c3);plot([0 1 1 0 0],[0 0 1 1 0]);disp('Mux');
  dotprod1 : neural/Weight Functions/dotprod
  dotprod2 : neural/Weight Functions/dotprod
  "lz{7,6}" : Outport
      mask Display: e = 0.06;c1 = [120 230 180]/255;c2 = ([120 230 180]+0)/(256+128);c3 = ([120 230 180]+128)/(256+128);patch([0 1 1 0],[0 0 1 1],c1);patch([0 1 1 1-e 1-e 0+e],[0 0 1 1-e 0+e 0+e],c2);patch([0 0 1 1-e 0+e 0+e],[0 1 1 1-e 1-e 0+e],c3);plot([0 1 1 0 0],[0 0 1 1 0]);
  wires:
  "IW{7,6}(1,:)'"/1 -> dotprod1/1
  "ad{7,6}"/1 -> dotprod1/2, dotprod2/2
  dotprod1/1 -> Mux/1
  "IW{7,6}(2,:)'"/1 -> dotprod2/1
  dotprod2/1 -> Mux/2
  Mux/1 -> "lz{7,6}"/1
